simulink model "COM_ViconController_x4morf_quat_withRecov_posMod"  (Simulink 8.6)
settings: Solver=FixedStepDiscrete  StartTime=0.0  StopTime=inf  FixedStep=ComMinSampleTime  RelTol=1e-3
values from neighbouring files (symbols this model uses):
  a_PWM = (MaxThrottle-MinThrottle)/(omega_r_max-omega_r_min)    [RobotParameters.m]
  b_PWM = MinThrottle - a_PWM*omega_r_min    [RobotParameters.m]
  BiasAcc = [-0.0791 0.072 -0.1481]    [AccCalib_Transformation_X4morf_Robot.mat]
  ComMinSampleTime = 1/400    (= 0.0025)    [init_ViconController_x4morf_quat_withRecov_posMod.m]
  dc_close = 25    [RobotParameters.m]
  dc_open = 63    [RobotParameters.m]
  g = 9.81    [RobotParameters.m]    (also in init_ViconController_x4morf_quat_withRecov_posMod.m)
  gamma_max = 89    [RobotParameters.m]
  LandingHeight = 0.08    [init_ViconController_x4morf_quat_withRecov_posMod.m]
  m = 0.380    (= 0.38)    [RobotParameters.m]
  MaxThrottle = 2000    [RobotParameters.m]
  MinThrottle = 1200    [RobotParameters.m]
  PositionSecuMax = [5.5 ; 3 ; 4]    [RobotParameters.m]
  PositionSecuMin = [-0.5; -3; -0.07]    [RobotParameters.m]
  Tacc = [0.9812  -0.03737  -0.0078; 0.0368  0.9984  -0.0083; 0.0232  -0.0002  0.9804]    [AccCalib_Transformation_X4morf_Robot.mat]
  time_unfolding = 230e-3    (= 0.23)    [RobotParameters.m]
  Tmax = .1643    (= 0.1643)    [RobotParameters.m]
  Tmin = .0183    (= 0.0183)    [RobotParameters.m]
  TorquesSat = zeros(3,181)    [gen_iGamma.m]
  Ts_AttitudeLoop = 1/200    (= 0.005)    [init_ViconController_x4morf_quat_withRecov_posMod.m]
  Ts_PositionLoop = 1/100    (= 0.01)    [init_ViconController_x4morf_quat_withRecov_posMod.m]
  Velocity_0 = [Vx_0 Vy_0 Vz_0]    [RobotParameters.m]
undefined symbols (not defined in the file or in its folder): DiscIntNeverNeededParam, Gumstix, MPU6050, UAVstruct
undefined symbols (not defined in the file): AccMax, AccMaxScenario, AccMin, AccMinScenario, b_est0, PositionMax, PositionMin, SpeedMax, SpeedMaxScenario, SpeedMin, SpeedMinScenario, Ts_Wifi
libraries: simulink x40, simulink_extras x11
(part 3 of 3)

== system COM_ViconController_x4morf_quat_withRecov_posMod/GUMSTIX/Positioning Mode/Vicon Position  Controller/PositionController1/PDX ==
  Pos_ref : Inport
  Pos_mes : Inport  Port=2
  S_ref : Inport  Port=3
  S_mes : Inport  Port=4
  Kp : Inport  Port=5
  Kd : Inport  Port=6
  Ki : Inport  Port=7
  Tf_int : Inport  Port=8
  Int_reset : Inport  Port=9
  Add : Sum  Inputs=+++
  Add1 : Sum  Inputs=+-
  Add2 : Sum  Inputs=+-
  Discrete filter first_ordrer1 : Subsystem
  Discrete-Time Integrator1 : DiscreteIntegrator  ExternalReset=level  SampleTime=-1  LimitOutput=on  UpperSaturationLimit=Max_Sat  LowerSaturationLimit=Min_Sat  ICPrevOutput=DiscIntNeverNeededParam  ICPrevScaledInput=DiscIntNeverNeededParam
  Mux : Mux  Inputs=5
  Product : Product  RndMeth=Zero
  Product1 : Product  RndMeth=Zero
  Product2 : Product  RndMeth=Zero
  cmd_sat : Outport
  X_PIDterm : Outport  Port=2
  wires:
  Tf_int/1 -> Discrete filter first_ordrer1/2(z0)
  Discrete filter first_ordrer1/1(y) -> Discrete-Time Integrator1/1
  Product1/1 -> Discrete filter first_ordrer1/1(u)
  Pos_mes/1 -> Add2/2
  Add2/1 -> Mux/1, Product/1
  Pos_ref/1 -> Add2/1
  Kp/1 -> Product/2
  Product/1 -> Mux/3, Add/1, Product1/1
  Kd/1 -> Product2/2
  S_ref/1 -> Add1/1
  S_mes/1 -> Add1/2
  Add1/1 -> Mux/2, Product2/1
  Product2/1 -> Mux/5, Add/3
  Ki/1 -> Product1/2
  Discrete-Time Integrator1/1 -> Mux/4, Add/2
  Int_reset/1 -> Discrete-Time Integrator1/2
  Add/1 -> cmd_sat/1
  Mux/1 -> X_PIDterm/1

== system COM_ViconController_x4morf_quat_withRecov_posMod/GUMSTIX/Positioning Mode/Vicon Position  Controller/PositionController1/PDY ==
  Pos_ref : Inport
  Pos_mes : Inport  Port=2
  S_ref : Inport  Port=3
  S_mes : Inport  Port=4
  Kp : Inport  Port=5
  Kd : Inport  Port=6
  Ki : Inport  Port=7
  Tf_int : Inport  Port=8
  Int_reset : Inport  Port=9
  Add : Sum  Inputs=+++
  Add1 : Sum  Inputs=+-
  Add2 : Sum  Inputs=+-
  Discrete filter first_ordrer1 : Subsystem
  Discrete-Time Integrator1 : DiscreteIntegrator  ExternalReset=level  SampleTime=-1  LimitOutput=on  UpperSaturationLimit=Max_Sat  LowerSaturationLimit=Min_Sat  ICPrevOutput=DiscIntNeverNeededParam  ICPrevScaledInput=DiscIntNeverNeededParam
  Mux : Mux  Inputs=5
  Product : Product  RndMeth=Zero
  Product1 : Product  RndMeth=Zero
  Product2 : Product  RndMeth=Zero
  cmd_sat : Outport
  Y_PIDterm : Outport  Port=2
  wires:
  Int_reset/1 -> Discrete-Time Integrator1/2
  Ki/1 -> Product1/2
  Add1/1 -> Mux/2, Product2/1
  S_mes/1 -> Add1/2
  S_ref/1 -> Add1/1
  Kd/1 -> Product2/2
  Kp/1 -> Product/2
  Pos_ref/1 -> Add2/1
  Add2/1 -> Mux/1, Product/1
  Pos_mes/1 -> Add2/2
  Product1/1 -> Discrete filter first_ordrer1/1(u)
  Discrete filter first_ordrer1/1(y) -> Discrete-Time Integrator1/1
  Tf_int/1 -> Discrete filter first_ordrer1/2(z0)
  Add/1 -> cmd_sat/1
  Product/1 -> Mux/3, Product1/1, Add/1
  Product2/1 -> Mux/5, Add/3
  Discrete-Time Integrator1/1 -> Mux/4, Add/2
  Mux/1 -> Y_PIDterm/1

== system COM_ViconController_x4morf_quat_withRecov_posMod/GUMSTIX/Positioning Mode/Vicon Position  Controller/PositionController1/PDZ ==
  Pos_ref : Inport
  Pos_mes : Inport  Port=2
  S_ref : Inport  Port=3
  S_mes : Inport  Port=4
  Kp : Inport  Port=5
  Kd : Inport  Port=6
  Ki : Inport  Port=7
  Tf_int : Inport  Port=8
  Int_reset : Inport  Port=9
  Add : Sum  Inputs=+++
  Add1 : Sum  Inputs=+-
  Add2 : Sum  Inputs=+-
  Discrete filter first_ordrer1 : Subsystem
  Discrete-Time Integrator1 : DiscreteIntegrator  ExternalReset=level  SampleTime=-1  LimitOutput=on  UpperSaturationLimit=Max_Sat*0.5  LowerSaturationLimit=-Max_Sat*0.5  ICPrevOutput=DiscIntNeverNeededParam  ICPrevScaledInput=DiscIntNeverNeededParam
  Mux : Mux  Inputs=5
  Product : Product  RndMeth=Zero
  Product1 : Product  RndMeth=Zero
  Product2 : Product  RndMeth=Zero
  cmd_sat : Outport
  Z_PIDterm : Outport  Port=2
  wires:
  Pos_mes/1 -> Add2/2
  Add2/1 -> Mux/1, Product/1
  Pos_ref/1 -> Add2/1
  Kp/1 -> Product/2
  Kd/1 -> Product2/2
  S_ref/1 -> Add1/1
  S_mes/1 -> Add1/2
  Add1/1 -> Mux/2, Product2/1
  Ki/1 -> Product1/2
  Int_reset/1 -> Discrete-Time Integrator1/2
  Tf_int/1 -> Discrete filter first_ordrer1/2(z0)
  Discrete filter first_ordrer1/1(y) -> Discrete-Time Integrator1/1
  Product1/1 -> Discrete filter first_ordrer1/1(u)
  Add/1 -> cmd_sat/1
  Product/1 -> Mux/3, Product1/1, Add/1
  Product2/1 -> Mux/5, Add/3
  Discrete-Time Integrator1/1 -> Mux/4, Add/2
  Mux/1 -> Z_PIDterm/1

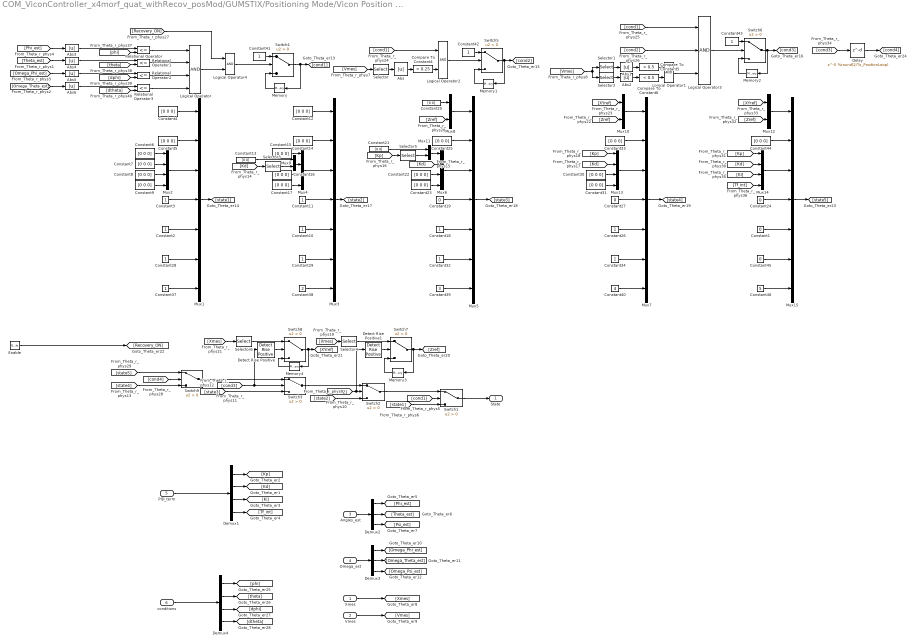
== system COM_ViconController_x4morf_quat_withRecov_posMod/GUMSTIX/Positioning Mode/Vicon Position  Controller/Recovery state machine/State machine ==
  Xmes : Inport
  Vmes : Inport  Port=2
  Angles_est : Inport  Port=3
  Omega_est : Inport  Port=4
  PID_term : Inport  Port=5
  conditions : Inport  Port=6
  Enable : EnablePort  StatesWhenEnabling=reset  ShowOutputPort=on
  Abs{,1..6} (7 alike) : Abs
  Compare To Constant4 : simulink/Logic and Bit Operations/Compare To Constant  relop=<  const=0.25  OutDataTypeStr=boolean
  Compare To Constant5 : simulink/Logic and Bit Operations/Compare To Constant  relop=<  const=0.5  OutDataTypeStr=boolean
  Compare To Constant6 : simulink/Logic and Bit Operations/Compare To Constant  relop=<  const=0.5  OutDataTypeStr=boolean
  Constant{1,19,24,27,45} (5 alike) : Constant  Value=0  OutDataTypeStr=Inherit: Inherit via back propagation
  Constant{2..3,10..11,18,26,28..29,32,34,37,41..43} (14 alike) : Constant  OutDataTypeStr=Inherit: Inherit via back propagation
  Constant{4..9,12,14..17,22..23,25,30..31,33,44} (18 alike) : Constant  Value=[0 0 0]  OutDataTypeStr=Inherit: Inherit via back propagation
  Constant13 : Constant  Value=[0 0]  OutDataTypeStr=Inherit: Inherit via back propagation
  Constant20 : Constant  Value=[0 0]  OutDataTypeStr=Inherit: Inherit via back propagation
  Constant21 : Constant  Value=[0 0]  OutDataTypeStr=Inherit: Inherit via back propagation
  Constant38 : Constant  Value=2  OutDataTypeStr=Inherit: Inherit via back propagation
  Constant39 : Constant  Value=3  OutDataTypeStr=Inherit: Inherit via back propagation
  Constant40 : Constant  Value=4  OutDataTypeStr=Inherit: Inherit via back propagation
  Constant46 : Constant  Value=5  OutDataTypeStr=Inherit: Inherit via back propagation
  Delay : Delay  DelayLength=5 %round(2/Ts_PositionLoop)  InitialCondition=0  SampleTime=Ts_PositionLoop
  Demux1 : Demux
  Demux2 : Demux  Outputs=3
  Demux3 : Demux  Outputs=3
  Demux4 : Demux
  Detect Rise Positive : simulink/Logic and Bit Operations/Detect Rise Positive  vinit=0  InputProcessing=Inherited  OutDataTypeStr=boolean
  Detect Rise Positive1 : simulink/Logic and Bit Operations/Detect Rise Positive  vinit=0  InputProcessing=Inherited  OutDataTypeStr=boolean
  Logical Operator : Logic  Inputs=4  AllPortsSameDT=off  OutDataTypeStr=boolean
  Logical Operator1 : Logic  AllPortsSameDT=off  OutDataTypeStr=boolean
  Logical Operator2 : Logic  AllPortsSameDT=off  OutDataTypeStr=boolean
  Logical Operator3 : Logic  Inputs=3  AllPortsSameDT=off  OutDataTypeStr=boolean
  Logical Operator4 : Logic  AllPortsSameDT=off  OutDataTypeStr=boolean
  Memory{,1..4} (5 alike) : Memory  InheritSampleTime=on
  Mux{1,3,5,7,15} (5 alike) : Mux  Inputs=7
  Mux{8..12} (5 alike) : Mux  Inputs=2
  Mux{2,4,6,13..14} (5 alike) : Mux
  Relational Operator{,1..3} (4 alike) : RelationalOperator  Operator=<=  OutDataTypeStr=boolean
  Selector{,3..5} (4 alike) : Selector  InputPortWidth=3  IndexOptions=Index vector (dialog)  Indices=[3]  OutputSizes=1
  Selector1 : Selector  InputPortWidth=3  IndexOptions=Index vector (dialog)  Indices=[1]  OutputSizes=1
  Selector2 : Selector  InputPortWidth=3  IndexOptions=Index vector (dialog)  Indices=[2]  OutputSizes=1
  Selector6 : Selector  InputPortWidth=3  IndexOptions=Index vector (dialog)  Indices=[1 2]  OutputSizes=1
  Switch{1..9} (9 alike) : Switch  Criteria=u2 > Threshold
  State : Outport  OutputWhenDisabled=reset  InitialOutput=1
  wires:
  Mux2/1 -> Mux1/3
  Constant2/1 -> Mux1/5
  Constant3/1 -> Mux1/4
  Constant6/1 -> Mux2/1
  Constant7/1 -> Mux2/2
  Constant8/1 -> Mux2/3
  Constant9/1 -> Mux2/4
  Constant4/1 -> Mux1/1
  Constant5/1 -> Mux1/2
  [Phi_est] -> Abs3/1
  [Theta_est] -> Abs4/1
  [Omega_Phi_est] -> Abs5/1
  [Omega_Theta_est] -> Abs6/1
  Relational Operator/1 -> Logical Operator/1
  Relational Operator1/1 -> Logical Operator/2
  Relational Operator2/1 -> Logical Operator/3
  Relational Operator3/1 -> Logical Operator/4
  [cond1] -> Switch1/2
  Mux1/1 -> [state1]
  [state1] -> Switch1/3
  Switch1/1 -> State/1
  [Vmes] -> Selector/1
  Selector/1 -> Abs/1
  Abs/1 -> Compare To Constant4/1
  [Vmes] -> Selector1/1, Selector2/1
  Selector2/1 -> Abs2/1
  Compare To Constant5/1 -> Logical Operator1/1
  Compare To Constant6/1 -> Logical Operator1/2
  Selector1/1 -> Abs1/1
  Abs1/1 -> Compare To Constant5/1
  Abs2/1 -> Compare To Constant6/1
  [cond2] -> Detect Rise Positive1/1, Switch2/2
  Switch2/1 -> Switch1/1
  [state2] -> Switch2/3
  [cond3] -> Detect Rise Positive/1, Switch3/2
  [state3] -> Switch3/3
  Switch3/1 -> Switch2/1
  Switch9/1 -> Switch3/1
  Mux4/1 -> Mux3/3
  Constant10/1 -> Mux3/5
  Constant11/1 -> Mux3/4
  Constant15/1 -> Mux4/1
  Mux9/1 -> Mux4/2
  Constant16/1 -> Mux4/3
  Constant17/1 -> Mux4/4
  Constant12/1 -> Mux3/1
  Constant14/1 -> Mux3/2
  Mux3/1 -> [state2]
  Constant18/1 -> Mux5/5
  Constant19/1 -> Mux5/4
  Constant25/1 -> Mux5/2
  Mux5/1 -> [state3]
  Constant26/1 -> Mux7/5
  Constant27/1 -> Mux7/4
  Constant33/1 -> Mux7/2
  Mux7/1 -> [state4]
  [Kd] -> Selector3/1
  Constant13/1 -> Mux9/1
  Selector3/1 -> Mux9/2
  Mux6/1 -> Mux5/3
  Mux11/1 -> Mux6/1
  [Kd] -> Mux6/2
  Constant22/1 -> Mux6/3
  Constant23/1 -> Mux6/4
  [Kp] -> Selector5/1
  Constant21/1 -> Mux11/1
  Selector5/1 -> Mux11/2
  Mux13/1 -> Mux7/3
  [Kp] -> Mux13/1
  [Kd] -> Mux13/2
  Constant30/1 -> Mux13/3
  Constant31/1 -> Mux13/4
  Mux8/1 -> Mux5/1
  Constant20/1 -> Mux8/1
  [Xmes] -> Selector4/1
  [Zref] -> Mux8/2
  Switch8/1 -> Memory4/1, [XYref]
  [Xmes] -> Selector6/1
  Mux10/1 -> Mux7/1
  [XYref] -> Mux10/1
  [Zref] -> Mux10/2
  Constant28/1 -> Mux1/6
  Constant29/1 -> Mux3/6
  Constant32/1 -> Mux5/6
  Constant34/1 -> Mux7/6
  Compare To Constant4/1 -> Logical Operator2/2
  Logical Operator1/1 -> Logical Operator3/3
  [cond1] -> Logical Operator3/1
  Abs5/1 -> Relational Operator2/1
  Abs6/1 -> Relational Operator3/1
  Constant37/1 -> Mux1/7
  Constant38/1 -> Mux3/7
  Constant39/1 -> Mux5/7
  Constant40/1 -> Mux7/7
  Logical Operator/1 -> Logical Operator4/2
  Memory1/1 -> Switch5/3
  Switch5/1 -> [cond2], Memory1/1
  Logical Operator2/1 -> Switch5/2
  Constant42/1 -> Switch5/1
  Memory2/1 -> Switch6/3
  Switch6/1 -> [cond3], Memory2/1
  Logical Operator3/1 -> Switch6/2
  Constant43/1 -> Switch6/1
  Memory3/1 -> Switch7/3
  Switch7/1 -> [Zref], Memory3/1
  Selector4/1 -> Switch7/1
  Memory4/1 -> Switch8/3
  Selector6/1 -> Switch8/1
  Detect Rise Positive/1 -> Switch8/2
  Detect Rise Positive1/1 -> Switch7/2
  Demux1/1 -> [Kp]
  Demux1/2 -> [Kd]
  Demux1/3 -> [Ki]
  Demux1/4 -> [Tf_int]
  PID_term/1 -> Demux1/1
  Angles_est/1 -> Demux2/1
  Demux2/1 -> [Phi_est]
  Demux2/2 -> [Theta_est]
  Demux2/3 -> [Psi_est]
  Xmes/1 -> [Xmes]
  Vmes/1 -> [Vmes]
  Omega_est/1 -> Demux3/1
  Demux3/1 -> [Omega_Phi_est]
  Demux3/2 -> [Omega_Theta_est]
  Demux3/3 -> [Omega_Psi_est]
  Enable/1 -> [Recovery_ON]
  [cond1] -> Logical Operator2/1
  [Recovery_ON] -> Logical Operator4/1
  [cond2] -> Logical Operator3/2
  Memory/1 -> Switch4/3
  Logical Operator4/1 -> Switch4/2
  Constant41/1 -> Switch4/1
  Switch4/1 -> Memory/1, [cond1]
  [state4] -> Switch9/3
  [cond4] -> Switch9/2
  [state5] -> Switch9/1
  Constant1/1 -> Mux15/5
  Constant24/1 -> Mux15/4
  Constant44/1 -> Mux15/2
  Mux15/1 -> [state5]
  Mux14/1 -> Mux15/3
  [Kp] -> Mux14/1
  [Kd] -> Mux14/2
  [Ki] -> Mux14/3
  [Tf_int] -> Mux14/4
  Mux12/1 -> Mux15/1
  [XYref] -> Mux12/1
  [Zref] -> Mux12/2
  Constant45/1 -> Mux15/6
  Constant46/1 -> Mux15/7
  [cond3] -> Delay/1
  Delay/1 -> [cond4]
  conditions/1 -> Demux4/1
  Demux4/1 -> [phi]
  Demux4/2 -> [theta]
  Demux4/3 -> [dphi]
  Demux4/4 -> [dtheta]
  Abs3/1 -> Relational Operator/1
  [phi] -> Relational Operator/2
  [theta] -> Relational Operator1/2
  Abs4/1 -> Relational Operator1/1
  [dphi] -> Relational Operator2/2
  [dtheta] -> Relational Operator3/2

== system COM_ViconController_x4morf_quat_withRecov_posMod/GUMSTIX/Positioning Mode/Vicon Position  Controller/PositionController1/PDX/Discrete filter first_ordrer1 ==
  u : Inport
  z0 : Inport  Port=2
  Add : Sum  Inputs=+-
  Add1 : Sum
  Constant : Constant  OutDataTypeStr=Inherit: Inherit via back propagation
  Divide : Product  Inputs=**
  Divide1 : Product  Inputs=**
  Memory : Memory  InheritSampleTime=on
  y : Outport
  wires:
  Constant/1 -> Add/1
  z0/1 -> Add/2, Divide/1
  Memory/1 -> Divide/2
  Add/1 -> Divide1/2
  u/1 -> Divide1/1
  Add1/1 -> Memory/1, y/1
  Divide1/1 -> Add1/1
  Divide/1 -> Add1/2

== system COM_ViconController_x4morf_quat_withRecov_posMod/GUMSTIX/Positioning Mode/Vicon Position  Controller/PositionController1/PDY/Discrete filter first_ordrer1 ==
  u : Inport
  z0 : Inport  Port=2
  Add : Sum  Inputs=+-
  Add1 : Sum
  Constant : Constant  OutDataTypeStr=Inherit: Inherit via back propagation
  Divide : Product  Inputs=**
  Divide1 : Product  Inputs=**
  Memory : Memory  InheritSampleTime=on
  y : Outport
  wires:
  Divide/1 -> Add1/2
  Divide1/1 -> Add1/1
  Add1/1 -> y/1, Memory/1
  u/1 -> Divide1/1
  Add/1 -> Divide1/2
  Memory/1 -> Divide/2
  z0/1 -> Divide/1, Add/2
  Constant/1 -> Add/1

== system COM_ViconController_x4morf_quat_withRecov_posMod/GUMSTIX/Positioning Mode/Vicon Position  Controller/PositionController1/PDZ/Discrete filter first_ordrer1 ==
  u : Inport
  z0 : Inport  Port=2
  Add : Sum  Inputs=+-
  Add1 : Sum
  Constant : Constant  OutDataTypeStr=Inherit: Inherit via back propagation
  Divide : Product  Inputs=**
  Divide1 : Product  Inputs=**
  Memory : Memory  InheritSampleTime=on
  y : Outport
  wires:
  Divide/1 -> Add1/2
  Divide1/1 -> Add1/1
  Add1/1 -> y/1, Memory/1
  u/1 -> Divide1/1
  Add/1 -> Divide1/2
  Memory/1 -> Divide/2
  z0/1 -> Divide/1, Add/2
  Constant/1 -> Add/1

== matlab function GUMSTIX/ESTIMATOR/Complementary Filter Quaternion gyro, acc, vicon GUMSTIX/Attitude_Est ==
  data: Q_hat_prec input single size=[4,1]; b_hat_prec input single size=[3,1]; gyro_imu input single size=[3,1]; acc_imu input single size=[3,1]; Q_Vicon input single size=[4,1]; dt input single size=1; k_a input single size=3; Q_hat output single size=[4,1]; b_hat output single size=[3,1]; Omega_hat output single size=[3, 1]; k_v input single size=3; k_b input single size=3; acc_ref input single size=3
function [Q_hat, b_hat, Omega_hat] = estimate_Complementary_Filter(Q_hat_prec, b_hat_prec, gyro_imu, acc_imu, Q_Vicon, dt, k_a, k_v, k_b, acc_ref)
    
    %#codegen
    
    
    % calculate the skew symetric matrix of the debiased gyro data
    Omega_hat = gyro_imu-b_hat_prec;
    
    % calculate the weighted correction 
    Q_tilde = QuaternionProduct(InvQuaternion(Q_Vicon), Q_hat_prec);
    s_tilde = Q_tilde(1);
    v_tilde = Q_tilde(2:4);
    
    alpha =    1/(norm(acc_ref)^2)*k_a.*cross(QuaternionVectorProduct(InvQuaternion(Q_hat_prec), acc_ref), acc_imu)...
             + k_v.*(s_tilde*v_tilde);
    
    % Construct the correction quaternion
    Q_corr = [        0        ;...
              Omega_hat - alpha];
    
    % determine the derivative of the rotation matrix
    dQ_hat = 0.5*QuaternionProduct(Q_hat_prec, Q_corr);
    % determine the derivative of the gyro's bias
    db_hat =k_b.*alpha;
    
    % First order Euler integration
    Q_hat = Q_hat_prec + dQ_hat*dt;
    
    % projection of the corrected quaternion (updated estimation of
    % attitude) onto Q
    Q_hat = UnitQuaternion(Q_hat);
    
    % time integration of the rotation matrix (euler forward)
    b_hat = b_hat_prec + db_hat*dt;
    
end

== matlab function GUMSTIX/Attitude controller/CTL_ATT_NL/Quaternion 2 Euler ==
  data: Q_hat input double; phi_hat output double; theta_hat output double; psi_hat output double
function [phi_hat, theta_hat, psi_hat] = rot2rad(Q_hat)
    
    %#codegen
    
    [phi_hat, theta_hat, psi_hat] = Quaternion2Euler(Q_hat);

end

== matlab function GUMSTIX/ESTIMATOR/MakeAngleContinous ==
  data: PsiEst input single; PsiCorr output single; PsiEst_prec input single; Offset_prec input single; Offset output single
function [PsiCorr, Offset] = MakeAngleContinous(PsiEst, PsiEst_prec, Offset_prec)
    %#codegen

    if(PsiEst_prec-PsiEst > pi)
        Offset = Offset_prec+2*pi;
        
    elseif (PsiEst_prec-PsiEst < -pi)
        Offset = Offset_prec-2*pi;
    else
        Offset = Offset_prec;   % do nothing
    end
    PsiCorr = PsiEst + Offset;
    
end

== matlab function GUMSTIX/Torques Disturbances/Triggered Subsystem/MATLAB Function ==
  data: TorquesDistMag input single; TorquesDist output single; Time input single; Dt input single
function TorquesDist = fcn(TorquesDistMag, Time, Dt)

    %#codegen
    
    TorquesDist = single(zeros(3,1));

    t1 = single(1);
    t2 = single(5);
    t3 = single(9);
    
    Dt = Dt/2;

    if (Time>=t1 && Time<t1+Dt)
        TorquesDist(1) = TorquesDistMag(1);
    elseif (Time>=t1+Dt && Time<t1+2*Dt)
        TorquesDist(1) = -TorquesDistMag(1);
    elseif (Time>=t2 && Time<t2+Dt)
        TorquesDist(2) = TorquesDistMag(2);
    elseif (Time>=t2+Dt && Time<t2+2*Dt)
        TorquesDist(2) = -TorquesDistMag(2);
    elseif (Time>=t3 && Time<t3+Dt)
        TorquesDist(3) = TorquesDistMag(3);
    elseif (Time>=t3+Dt && Time<t3+2*Dt)
        TorquesDist(3) = -TorquesDistMag(3);
    else
        % do nothing, all torques are null
    end

end

== matlab function GUMSTIX/Attitude controller/CTL_ATT_NL/AttCtrl Perso ==
  data: Q_ref input double size=[4, 1]; Torques output double size=[3, 1]; eR output double; Omega_ref output single size=[3,1]; Iterm output double; Dterm output double; Q_est input double size=[4, 1]; Omega_est input double size=[3, 1]; I input double size=[3, 3]; Komega_perso input double size=[3, 1]; Ktorques_perso input double size=[3, 1]; Kint_perso input double; dt input double; Pos input double; GyroTerm output double size=[3,1]; LandingHeight input double; cutIntXY input double; eI_prec input single; eI output single
function [Torques, eR, Omega_ref, Iterm, Dterm, GyroTerm, eI] = AttitudeController(Q_ref, Q_est, Omega_est, I, Komega_perso, Ktorques_perso, Kint_perso, dt, Pos, LandingHeight, cutIntXY, eI_prec)
    
    % calculate the Attitude error 
    Q_tilde = QuaternionProduct(InvQuaternion(Q_est), Q_ref);
%     s_tilde = 2*acos(Q_tilde(1));
%     v_tilde = Q_tilde(2:4)/sin(s_tilde/2);
    s_tilde = Q_tilde(1);
    v_tilde = Q_tilde(2:4);
    eR = s_tilde*v_tilde;
    
    if s_tilde >= 0
        Omega_ref = 2*diag(Komega_perso)*v_tilde;
    else
        Omega_ref = -2*diag(Komega_perso)*v_tilde;
    end
    
    eI = eI_prec;
    if Pos(3)>= LandingHeight && cutIntXY == 0
        eI = eI_prec + Kint_perso.*(eR*dt);
    elseif Pos(3)>= LandingHeight && cutIntXY == 1
        eI(1:2) = eI_prec(1:2);
        eI(3) = eI_prec(3) + Kint_perso(3).*(eR(3)*dt);
    end
    
    Dterm = I*diag(Ktorques_perso)*(Omega_ref-Omega_est);
    Iterm = I*eI;
    
    GyroTerm = single([0 0 0]'); % cross(Omega_est, I*Omega_est);
    
    Torques = Dterm + Iterm + GyroTerm;
end

== matlab function GUMSTIX/Torques Disturbances/Triggered Subsystem1/MATLAB Function ==
  data: TorquesDistMag input single; TorquesDist output single; Time input single; Dt input single
function TorquesDist = fcn(TorquesDistMag, Time, Dt)

    %#codegen
    
    TorquesDist = single(zeros(3,1));

    t1 = single(1);
    t2 = single(5);
    t3 = single(9);

    if (Time>=t1 && Time<t1+Dt)
        TorquesDist(1) = TorquesDistMag(1);
    elseif (Time>=t2 && Time<t2+Dt)
        TorquesDist(2) = TorquesDistMag(2);
    elseif (Time>=t3 && Time<t3+Dt)
        TorquesDist(3) = TorquesDistMag(3);
    else
        % do nothing, all torques are null
    end

end

== matlab function GUMSTIX/Attitude controller/CTL_ATT_NL/Euler 2 Quaternion1 ==
  data: angles input double; Q output double
function Q  = Euler2Quaternion(angles)
    
    Q = Euler2Quaternion(angles(1), angles(2), angles(3));

end

== matlab function GUMSTIX/Arena Security/MATLAB Function ==
  data: xyz input double size=3; secu_ON output double; PositionSecuMin parameter double size=3; PositionSecuMax parameter double size=3
function secu_ON = fcn(xyz, PositionSecuMin, PositionSecuMax)
%#codegen

x = xyz(1);
y = xyz(2);
z = xyz(3);

if ( x >= PositionSecuMax(1) || x <= PositionSecuMin(1) ||  y >= PositionSecuMax(2) || y <= PositionSecuMin(2) ||  z >= PositionSecuMax(3) || z <= PositionSecuMin(3) )
    secu_ON = 1;
else
    secu_ON = 0;
end

end

== matlab function GUMSTIX/Attitude controller/CTL_ATT_NL/Angles Disturbances/Triggered Subsystem/MATLAB Function ==
  data: AnglesDistMag input single; AnglesDist output single; Time input single; Dt input single
function AnglesDist = fcn(AnglesDistMag, Time, Dt)

    %#codegen
    
    AnglesDist = single(zeros(3,1));

    t1 = single(1);
    t2 = single(5);
    t3 = single(9);
    
    Dt = Dt/2;

    if (Time>=t1 && Time<t1+Dt)
        AnglesDist(1) = AnglesDistMag(1);
    elseif (Time>=t1+Dt && Time<t1+2*Dt)
        AnglesDist(1) = -AnglesDistMag(1);
    elseif (Time>=t2 && Time<t2+Dt)
        AnglesDist(2) = AnglesDistMag(2);
    elseif (Time>=t2+Dt && Time<t2+2*Dt)
        AnglesDist(2) = -AnglesDistMag(2);
    elseif (Time>=t3 && Time<t3+Dt)
        AnglesDist(3) = AnglesDistMag(3);
    elseif (Time>=t3+Dt && Time<t3+2*Dt)
        AnglesDist(3) = -AnglesDistMag(3);
    else
        % do nothing, all torques are null
    end

end

== matlab function GUMSTIX/Control Mix/Control_mix/Mixage ==
  data: iGamma input double; ThrustTorques input double; gamma input double; omega2 output double
function omega2 = mixage(iGamma,ThrustTorques,gamma)
% Inverse Gamma matrix
% INPUTS
%	- gamma :	folding angle		[deg]
% OUTPUTS
%	- omega2:	Rotor speed square	[rad]^2

omega2 = iGamma(:,:,gamma+1)*ThrustTorques;
		
end

== matlab function GUMSTIX/Torques saturation/MATLAB Function ==
  data: TorquesSat input double; gamma input double; TSat output double
function TSat = torque_select(TorquesSat,gamma)
% Select torque saturation (depends of gamma)

TSat = TorquesSat(:,gamma+1);

end

== matlab function GUMSTIX/ESTIMATOR/Quaternion 2 Euler ==
  data: Q_hat input double; phi_hat output double; theta_hat output double; psi_hat output double
function [phi_hat, theta_hat, psi_hat] = rot2rad(Q_hat)
    
    %#codegen
    
    [phi_hat, theta_hat, psi_hat] = Quaternion2Euler(Q_hat);

end

== matlab function GUMSTIX/Positioning Mode/Euler 2 Quaternion1 ==
  data: angles input double; Q output double
function Q  = Euler2Quaternion(angles)
    
    %#codegen
    Q = Euler2Quaternion(angles(1), angles(2), angles(3));

end
